simulink model "Termin2VE_changed"  (R2014a)
settings: Solver=ode3  StartTime=0.0  StopTime=16/8000  FixedStep=1/8000  RelTol=1e-3
undefined symbols (not defined in the file or in its folder): get
libraries: dspsnks4 x8, dspxfrm3 x4, dspsigops x3, dspsrcs4 x1
settings Model: Creator=dsv1_5  LastModifiedBy=dsv1_5

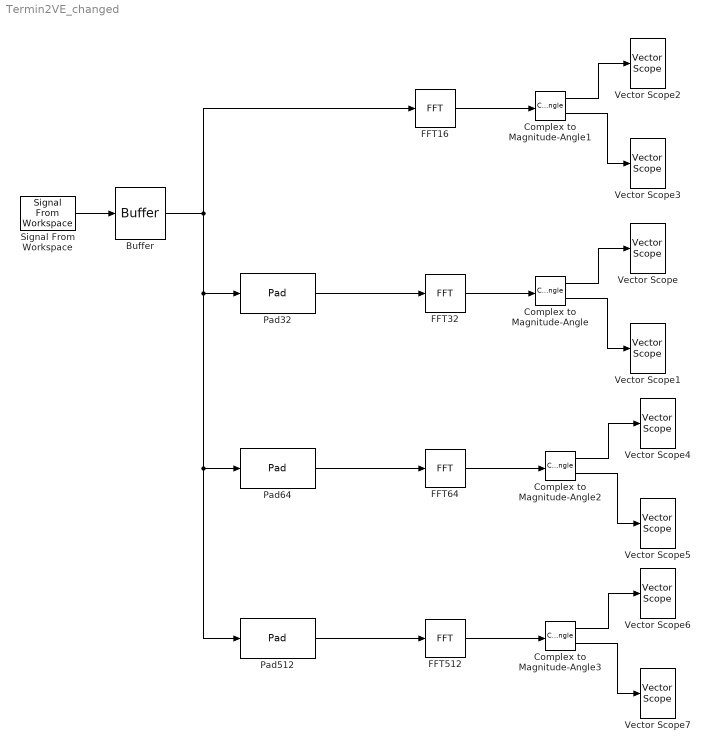
== system Termin2VE_changed ==
  Buffer : Buffer  N=16  TreatMby1Signals=One channel
  Complex to Magnitude-Angle{,1..3} (4 alike) : ComplexToMagnitudeAngle
  "FFT16 " : dspxfrm3/FFT  CompMethod=Table lookup  TableOpt=NEW  TableOptActive=Speed  BitRevOrder=off  InheritFFTLength=on  FFTLength=16  WrapInput=on  RowConvenienceOn=on  FFTImplementation=Auto  SkipNorm=off  firstCoeffDataTypeStr=Inherit: Same word length as input  firstCoeffLastDataTypeStr=Inherit: Same word length as input  outputMin=[]  outputMax=[]  roundingMode=Floor  overflowMode=off
  FFT32 : dspxfrm3/FFT  CompMethod=Table lookup  TableOpt=NEW  TableOptActive=Speed  BitRevOrder=off  InheritFFTLength=on  FFTLength=32  WrapInput=on  RowConvenienceOn=on  FFTImplementation=Auto  SkipNorm=off  firstCoeffDataTypeStr=Inherit: Same word length as input  firstCoeffLastDataTypeStr=Inherit: Same word length as input  outputMin=[]  outputMax=[]  roundingMode=Floor  overflowMode=off
  FFT512 : dspxfrm3/FFT  CompMethod=Table lookup  TableOpt=NEW  TableOptActive=Speed  BitRevOrder=off  InheritFFTLength=on  FFTLength=512  WrapInput=on  RowConvenienceOn=on  FFTImplementation=Auto  SkipNorm=off  firstCoeffDataTypeStr=Inherit: Same word length as input  firstCoeffLastDataTypeStr=Inherit: Same word length as input  outputMin=[]  outputMax=[]  roundingMode=Floor  overflowMode=off
  FFT64 : dspxfrm3/FFT  CompMethod=Table lookup  TableOpt=NEW  TableOptActive=Speed  BitRevOrder=off  InheritFFTLength=on  FFTLength=64  WrapInput=on  RowConvenienceOn=on  FFTImplementation=Auto  SkipNorm=off  firstCoeffDataTypeStr=Inherit: Same word length as input  firstCoeffLastDataTypeStr=Inherit: Same word length as input  outputMin=[]  outputMax=[]  roundingMode=Floor  overflowMode=off
  Pad32 : dspsigops/Pad  padAlong=Columns  dimsToPad=1  valSrc=Specify via dialog  padVal=0  spec=Output size  padNumOutRowsSpecMethod=User-specified  numOutRows=32  padNumOutColsSpecMethod=User-specified  numOutCols=1  isVarDimsMode=off  padBeginning=0  padEnd=0  outSizeMode=User-specified  outSize=1  padSigAt=End  trunc_flag=None  roundingMode=Floor  overflowMode=off  truncOrWrapMode=Truncate  wrap_flag=None
  Pad512 : dspsigops/Pad  padAlong=Columns  dimsToPad=1  valSrc=Specify via dialog  padVal=0  spec=Output size  padNumOutRowsSpecMethod=User-specified  numOutRows=512  padNumOutColsSpecMethod=User-specified  numOutCols=1  isVarDimsMode=off  padBeginning=0  padEnd=0  outSizeMode=User-specified  outSize=1  padSigAt=End  trunc_flag=None  roundingMode=Floor  overflowMode=off  truncOrWrapMode=Truncate  wrap_flag=None
  Pad64 : dspsigops/Pad  padAlong=Columns  dimsToPad=1  valSrc=Specify via dialog  padVal=0  spec=Output size  padNumOutRowsSpecMethod=User-specified  numOutRows=64  padNumOutColsSpecMethod=User-specified  numOutCols=1  isVarDimsMode=off  padBeginning=0  padEnd=0  outSizeMode=User-specified  outSize=1  padSigAt=End  trunc_flag=None  roundingMode=Floor  overflowMode=off  truncOrWrapMode=Truncate  wrap_flag=None
  Signal From Workspace : dspsrcs4/Signal From Workspace  X=signal1  Ts=1/8000  nsamps=1  OutputAfterFinalValue=Setting to zero  ignoreOrWarnInputAndFrameLengths=off
  Vector Scope{,1..7} (8 alike) : dspsnks4/Vector Scope  ScopeProperties=on  Domain=Time  HorizSpan=1  DisplayProperties=off  AxisGrid=on  Memory=off  FrameNumber=on  AxisLegend=off  AxisZoom=off  OpenScopeAtSimStart=on  OpenScopeImmediately=off  FigPos=get(0,'defaultfigureposition')  AxisProperties=off  XUnits=Hertz  XRange=[0...Fs/2]  InheritXIncr=on  XIncr=1  XLabel=Time  XLimit=Auto  XMin=0  XMax=1  XStart=0  YUnits=dB  YLabel=Amplitude  LineProperties=off  XAxisParamsVer=6.9
      settings: YMin=-10  YMax=10
  wires:
  Pad32/1 -> FFT32/1
  Signal From Workspace/1 -> Buffer/1
  Pad64/1 -> FFT64/1
  Pad512/1 -> FFT512/1
  Complex to Magnitude-Angle/1 -> Vector Scope/1
  Complex to Magnitude-Angle/2 -> Vector Scope1/1
  Buffer/1 -> Pad32/1, Pad64/1, Pad512/1, "FFT16 "/1
  FFT32/1 -> Complex to Magnitude-Angle/1
  Complex to Magnitude-Angle1/1 -> Vector Scope2/1
  Complex to Magnitude-Angle1/2 -> Vector Scope3/1
  "FFT16 "/1 -> Complex to Magnitude-Angle1/1
  Complex to Magnitude-Angle2/1 -> Vector Scope4/1
  Complex to Magnitude-Angle2/2 -> Vector Scope5/1
  FFT64/1 -> Complex to Magnitude-Angle2/1
  Complex to Magnitude-Angle3/1 -> Vector Scope6/1
  Complex to Magnitude-Angle3/2 -> Vector Scope7/1
  FFT512/1 -> Complex to Magnitude-Angle3/1
